simulink model "Ejemplo_neurosky"  (R2016a)
settings: Solver=FixedStepDiscrete  StartTime=0.0  StopTime=inf  FixedStep=1/512  RelTol=1e-3
libraries: LibrarySimulinkSAS x1, aerolibanimutils x1
settings Model: Creator=Usuario  LastModifiedBy=Usuario

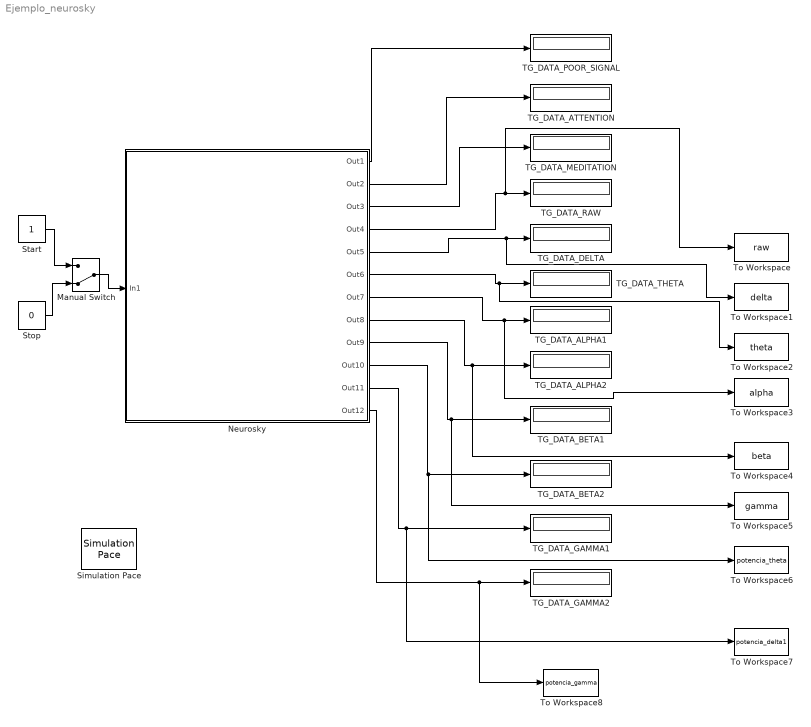
== system Ejemplo_neurosky ==
  Manual Switch : ManualSwitch  CurrentSetting=0
  Neurosky : Subsystem
      mask Display:
      | image('neurosky.jpg')
      | color('red')
      | port_label('input',1,'Start/Stop')
      | color('blue')
      | port_label('output',1,'POOR_SIGNAL')
      | port_label('output',2,'ATTENTION')
      | port_label('output',3,'MEDITATION')
      | port_label('output',4,'DATA RAW')
      | port_label('output',5,'DELTA')
      | port_label('output',6,'THETA')
      | port_label('output',7,'ALPHA1')
      | port_label('output',8,'ALPHA2')
      | port_label('output',9,'BETA1')
      | port_label('output',10,'BETA2')
      | port_label('output',11,'GAMMA1')
      | port_label('output',12,'GAMMA2')
  Simulation Pace : aerolibanimutils/Simulation Pace  SimulationPace=1  SleepMode=MATLAB Thread  OutputPaceError=off  SampleTime=-1
  Start : Constant  OutDataTypeStr=single
  Stop : Constant  Value=0  OutDataTypeStr=single
  TG_DATA_ALPHA1 : Display
  TG_DATA_ALPHA2 : Display
  TG_DATA_ATTENTION : Display
  TG_DATA_BETA1 : Display
  TG_DATA_BETA2 : Display
  TG_DATA_DELTA : Display
  TG_DATA_GAMMA1 : Display
  TG_DATA_GAMMA2 : Display
  TG_DATA_MEDITATION : Display
  TG_DATA_POOR_SIGNAL : Display
  TG_DATA_RAW : Display
  TG_DATA_THETA : Display
  To Workspace : ToWorkspace  VariableName=raw  SaveFormat=Structure With Time  SampleTime=-1
  To Workspace1 : ToWorkspace  VariableName=delta  SaveFormat=Structure With Time  SampleTime=-1
  To Workspace2 : ToWorkspace  VariableName=theta  SaveFormat=Structure With Time  SampleTime=-1
  To Workspace3 : ToWorkspace  VariableName=alpha  SaveFormat=Structure With Time  SampleTime=-1
  To Workspace4 : ToWorkspace  VariableName=beta  SaveFormat=Structure With Time  SampleTime=-1
  To Workspace5 : ToWorkspace  VariableName=gamma  SaveFormat=Structure With Time  SampleTime=-1
  To Workspace6 : ToWorkspace  VariableName=potencia_theta  SaveFormat=Structure With Time  SampleTime=-1
  To Workspace7 : ToWorkspace  VariableName=potencia_delta1  SaveFormat=Structure With Time  SampleTime=-1
  To Workspace8 : ToWorkspace  VariableName=potencia_gamma  SaveFormat=Structure With Time  SampleTime=-1
  wires:
  Neurosky/1(Out1) -> TG_DATA_POOR_SIGNAL/1
  Neurosky/2(Out2) -> TG_DATA_ATTENTION/1
  Neurosky/3(Out3) -> TG_DATA_MEDITATION/1
  Neurosky/4(Out4) -> To Workspace/1, TG_DATA_RAW/1
  Neurosky/5(Out5) -> To Workspace1/1, TG_DATA_DELTA/1
  Neurosky/6(Out6) -> To Workspace2/1, TG_DATA_THETA/1
  Neurosky/7(Out7) -> To Workspace3/1, TG_DATA_ALPHA1/1
  Neurosky/8(Out8) -> To Workspace4/1, TG_DATA_ALPHA2/1
  Neurosky/9(Out9) -> To Workspace5/1, TG_DATA_BETA1/1
  Neurosky/10(Out10) -> To Workspace6/1, TG_DATA_BETA2/1
  Neurosky/11(Out11) -> To Workspace7/1, TG_DATA_GAMMA1/1
  Neurosky/12(Out12) -> To Workspace8/1, TG_DATA_GAMMA2/1
  Stop/1 -> Manual Switch/2
  Start/1 -> Manual Switch/1
  Manual Switch/1 -> Neurosky/1(In1)

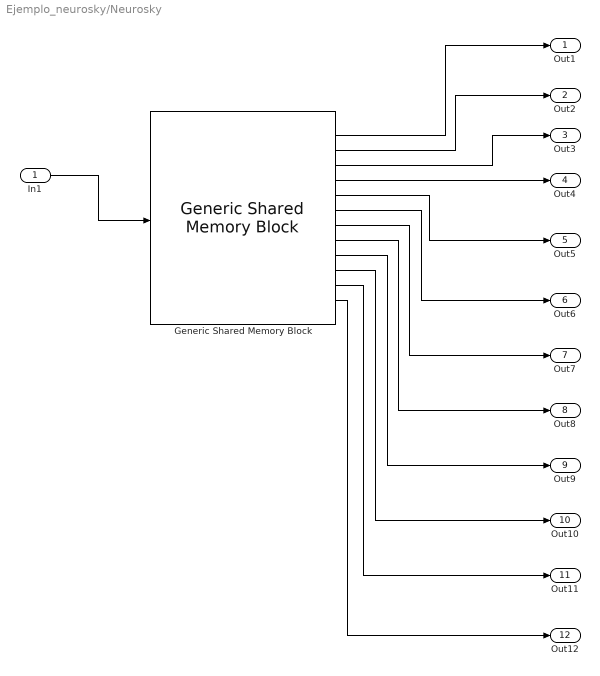
== system Ejemplo_neurosky/Neurosky ==
  In1 : Inport
  Generic Shared Memory Block : LibrarySimulinkSAS/Generic Shared Memory Block  nombre='NEUROSKY'  dispositivo=1  vecE=[1]  vecS=[1 1 1 1 1 1 1 1 1 1 1 1]  tipoE=['f']  tipoS=['f' 'f' 'f' 'f' 'f' 'f' 'f' 'f' 'f' 'f' 'f' 'f']
  Out1 : Outport
  Out2 : Outport  Port=2
  Out3 : Outport  Port=3
  Out4 : Outport  Port=4
  Out5 : Outport  Port=5
  Out6 : Outport  Port=6
  Out7 : Outport  Port=7
  Out8 : Outport  Port=8
  Out9 : Outport  Port=9
  Out10 : Outport  Port=10
  Out11 : Outport  Port=11
  Out12 : Outport  Port=12
  wires:
  Generic Shared Memory Block/3 -> Out3/1
  Generic Shared Memory Block/7 -> Out7/1
  Generic Shared Memory Block/9 -> Out9/1
  Generic Shared Memory Block/5 -> Out5/1
  Generic Shared Memory Block/8 -> Out8/1
  Generic Shared Memory Block/2 -> Out2/1
  Generic Shared Memory Block/11 -> Out11/1
  Generic Shared Memory Block/12 -> Out12/1
  Generic Shared Memory Block/10 -> Out10/1
  Generic Shared Memory Block/4 -> Out4/1
  Generic Shared Memory Block/6 -> Out6/1
  Generic Shared Memory Block/1 -> Out1/1
  In1/1 -> Generic Shared Memory Block/1
